simulink model "MadIot"  (R2022b)
settings: Solver=ode113  StartTime=0.0  StopTime=5  RelTol=1e-3
undefined symbols (not defined in the file): Discrete, linsys1, Time
libraries: spsThreePhaseVIMeasurementLib x46, spsThreePhasePISectionLineLib x20, spsThreePhaseSeriesRLCLoadLib x12, spsThreePhaseBreakerLib x7, spsThreePhaseTransformerTwoWindingsLib x5, ctrlSharedLib x3, spsThreePhaseDynamicLoadLib x3, spsSynchronousMachinepuStandardLib x3, spsThreePhaseParallelRLCLoadLib x3, spsExcitationSystemLib x3, spsGenericPowerSystemStabilizerLib x3, spsHydraulicTurbineandGovernorLib x3
(part 1 of 3)
settings Model: Creator=root  LastModifiedBy=suman
settings DataIOCC: SaveFormat=Array  SaveOutput=off  SignalLogging=off  DSMLogging=off  SaveTime=off  ReturnWorkspaceOutputs=off
settings DebuggingCC: UnconnectedInputMsg=warning  UnconnectedOutputMsg=warning  UnconnectedLineMsg=warning  SFMachineParentedDataDiag=warning  ArithmeticOperatorsInVariantConditions=warning
settings ModelReferenceCC: EnableRefExpFcnMdlSchedulingChecks=on
settings SFSimCC: CustomCodeUndefinedFunction=UseInterfaceOnly
settings RTWCC: DLArmComputeVersion=19.05

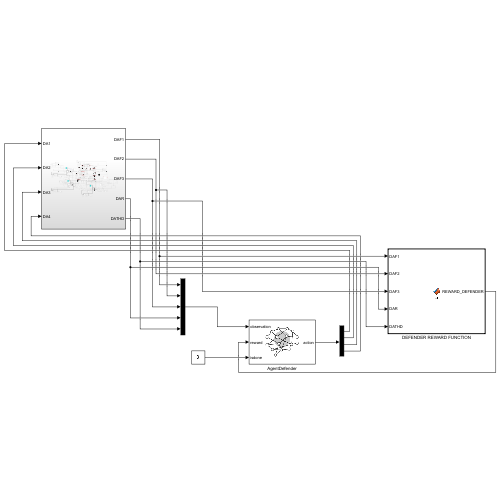
[thumbnail: Simulink's stored preview of the top-level diagram]
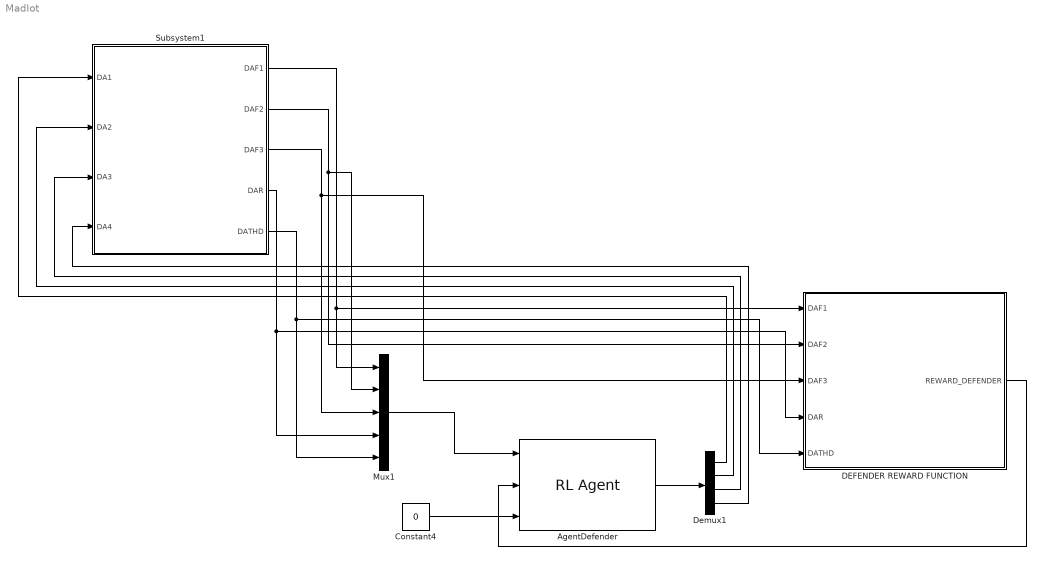
== system MadIot ==
  AgentDefender : rllib/RL Agent  Agent=AgentDefender_1  ExternalActionAsInput=off  ProvideLastAction=off  ProvideCumRwd=off  TreatAsDirectFeedthrough=on  UseStrictObservationDataTypes=off
  Constant4 : Constant  Value=0
  DEFENDER REWARD FUNCTION : MATLAB Function  TreatAsAtomicUnit=on
  Demux1 : Demux
  Mux1 : Mux  Inputs=5
  Subsystem1 : Subsystem
  wires:
  Subsystem1/1(DAF1) -> Mux1/1, DEFENDER REWARD FUNCTION/1(DAF1)
  Subsystem1/2(DAF2) -> DEFENDER REWARD FUNCTION/2(DAF2), Mux1/2
  Subsystem1/3(DAF3) -> DEFENDER REWARD FUNCTION/3(DAF3), Mux1/3
  Subsystem1/4(DAR) -> DEFENDER REWARD FUNCTION/4(DAR), Mux1/4
  Subsystem1/5(DATHD) -> DEFENDER REWARD FUNCTION/5(DATHD), Mux1/5
  Mux1/1 -> AgentDefender/1
  Constant4/1 -> AgentDefender/3
  Demux1/1 -> Subsystem1/1(DA1)
  Demux1/2 -> Subsystem1/2(DA2)
  Demux1/3 -> Subsystem1/3(DA3)
  Demux1/4 -> Subsystem1/4(DA4)
  AgentDefender/1 -> Demux1/1
  DEFENDER REWARD FUNCTION/1(REWARD_DEFENDER) -> AgentDefender/2
